simulink model "PID"  (R2022b)
settings: Solver=VariableStepAuto  StartTime=0.0  StopTime=30  RelTol=1e-3
InitFcn:
  | Kp = 10;
  | Ki = 2;
  | Kd = 1;
settings Model: Creator=user  LastModifiedBy=user

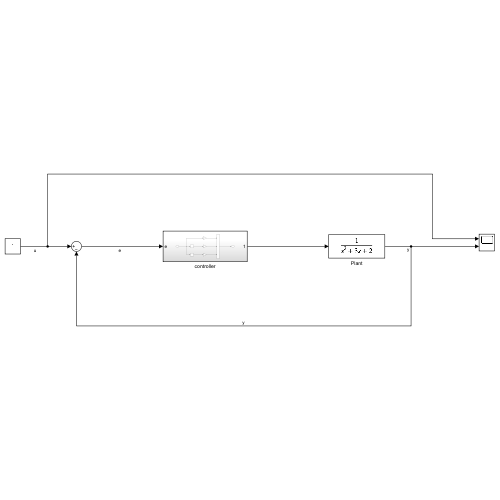
[thumbnail: Simulink's stored preview of the top-level diagram]
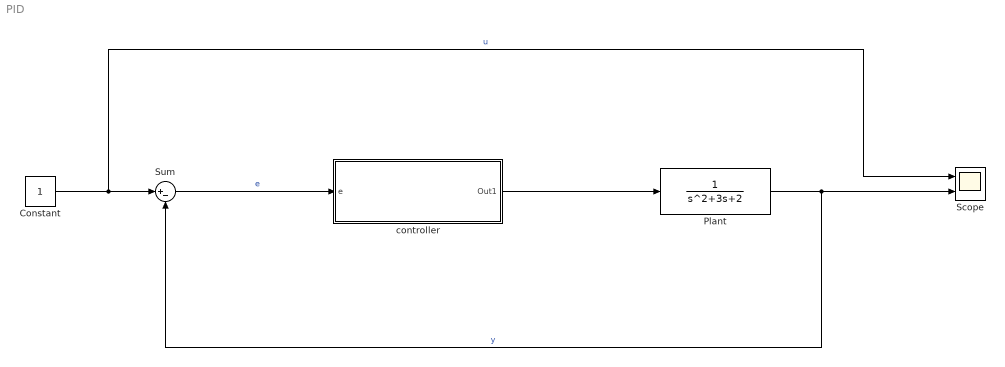
== system PID ==
  Constant : Constant
  Plant : TransferFcn  Denominator=[1 3 2]
  Scope : Scope  NumInputPorts=2
  Sum : Sum  Inputs=|+-
  controller : Subsystem
  wires:
  Plant/1 -> Sum/2, Scope/2  "y"
  Constant/1 -> Scope/1, Sum/1  "u"
  Sum/1 -> controller/1(e)  "e"
  controller/1(Out1) -> Plant/1

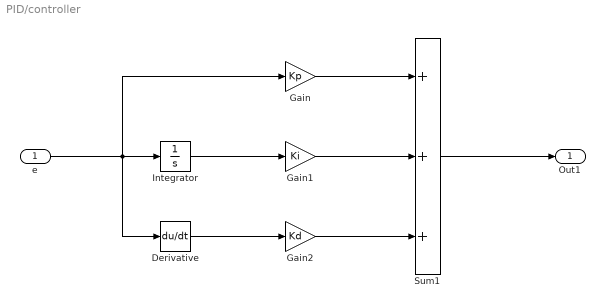
== system PID/controller ==
  e : Inport
  Derivative : Derivative
  Gain : Gain  Gain=Kp
  Gain1 : Gain  Gain=Ki
  Gain2 : Gain  Gain=Kd
  Integrator : Integrator
  Sum1 : Sum  Inputs=+++
  Out1 : Outport
  wires:
  Gain1/1 -> Sum1/2
  Gain/1 -> Sum1/1
  e/1 -> Derivative/1, Integrator/1, Gain/1
  Sum1/1 -> Out1/1
  Derivative/1 -> Gain2/1
  Gain2/1 -> Sum1/3
  Integrator/1 -> Gain1/1
